simulink model "Test_Sistema_piero"  (R2022b)
settings: Solver=VariableStepAuto  StartTime=0.0  StopTime=10.0  RelTol=1e-3
libraries: arduinolib x11, simulink x3
settings Model: Creator=marqu  LastModifiedBy=marqu

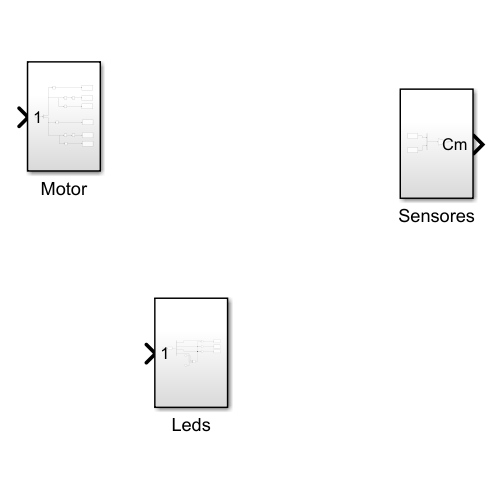
[thumbnail: Simulink's stored preview of the top-level diagram]
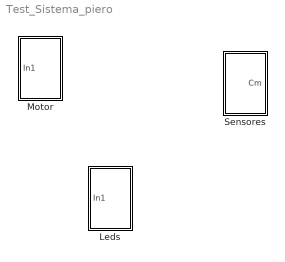
== system Test_Sistema_piero ==
  Leds : Subsystem
  Motor : Subsystem
  Sensores : Subsystem

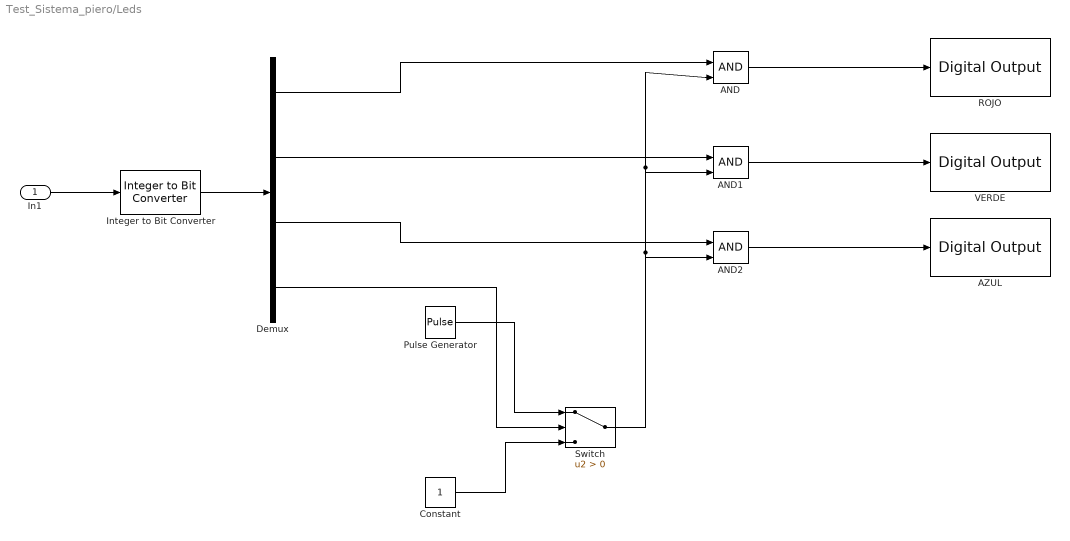
== system Test_Sistema_piero/Leds ==
  In1 : Inport
  AND : Logic  IconShape=distinctive  AllPortsSameDT=off  OutDataTypeStr=boolean
  AND1 : Logic  IconShape=distinctive  AllPortsSameDT=off  OutDataTypeStr=boolean
  AND2 : Logic  IconShape=distinctive  AllPortsSameDT=off  OutDataTypeStr=boolean
  AZUL : arduinolib/Digital Output  pinNumber=53  Direction=output  blockPlatform=arduino
  Constant : Constant
  Demux : Demux
  Integer to Bit Converter : simulink/Logic and Bit Operations/Integer to Bit Converter  nbits=3  signedInputValues=Unsigned  bitOrder=MSB first  outDtype=Inherit via internal rule
  Pulse Generator : DiscretePulseGenerator  PulseType=Time based  Period=10  PulseWidth=5
  ROJO : arduinolib/Digital Output  pinNumber=49  Direction=output  blockPlatform=arduino
  Switch : Switch  Criteria=u2 > Threshold  SaturateOnIntegerOverflow=off  InputSameDT=off
  VERDE : arduinolib/Digital Output  pinNumber=51  Direction=output  blockPlatform=arduino
  wires:
  AND1/1 -> VERDE/1
  Demux/4 -> Switch/2
  Integer to Bit Converter/1 -> Demux/1
  Constant/1 -> Switch/3
  Demux/3 -> AND2/1
  Demux/1 -> AND/1
  Demux/2 -> AND1/1
  Switch/1 -> AND2/2, AND1/2, AND/2
  AND2/1 -> AZUL/1
  In1/1 -> Integer to Bit Converter/1
  AND/1 -> ROJO/1
  Pulse Generator/1 -> Switch/1

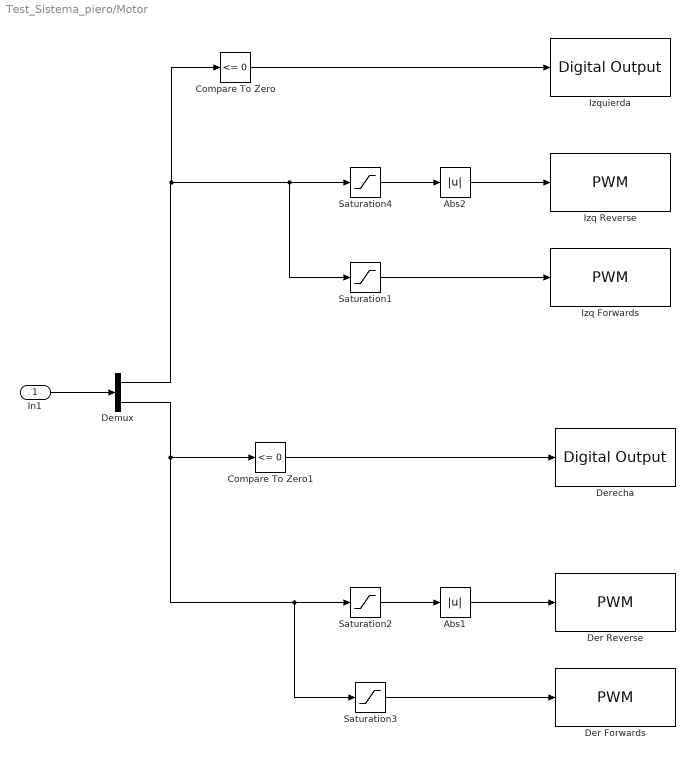
== system Test_Sistema_piero/Motor ==
  In1 : Inport
  Abs1 : Abs  SaturateOnIntegerOverflow=off
  Abs2 : Abs  SaturateOnIntegerOverflow=off
  Compare To Zero : simulink/Logic and Bit Operations/Compare To Zero  relop=<=  OutDataTypeStr=boolean
  Compare To Zero1 : simulink/Logic and Bit Operations/Compare To Zero  relop=<=  OutDataTypeStr=boolean
  Demux : Demux  Outputs=2
  Der Forwards : arduinolib/PWM  pinNumber=11  frequencyType=Default  desiredFrequency=490.2  achievableFrequency=490.2
  Der Reverse : arduinolib/PWM  pinNumber=12  frequencyType=Default  desiredFrequency=490.2  achievableFrequency=490.2
  Derecha : arduinolib/Digital Output  pinNumber=13  Direction=output  blockPlatform=arduino
  Izq Forwards : arduinolib/PWM  pinNumber=10  frequencyType=Default  desiredFrequency=490.2  achievableFrequency=490.2
  Izq Reverse : arduinolib/PWM  pinNumber=9  frequencyType=Default  desiredFrequency=490.2  achievableFrequency=490.2
  Izquierda : arduinolib/Digital Output  pinNumber=8  Direction=output  blockPlatform=arduino
  Saturation{1..4} (4 alike) : Saturate
  wires:
  In1/1 -> Demux/1
  Abs1/1 -> Der Reverse/1
  Compare To Zero1/1 -> Derecha/1
  Abs2/1 -> Izq Reverse/1
  Compare To Zero/1 -> Izquierda/1
  Demux/1 -> Compare To Zero/1, Saturation4/1, Saturation1/1
  Demux/2 -> Compare To Zero1/1, Saturation2/1, Saturation3/1
  Saturation3/1 -> Der Forwards/1
  Saturation4/1 -> Abs2/1
  Saturation1/1 -> Izq Forwards/1
  Saturation2/1 -> Abs1/1

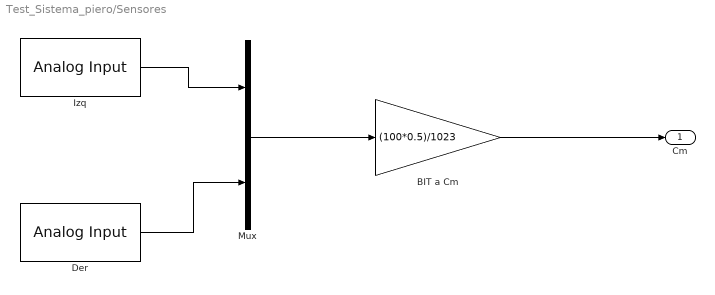
== system Test_Sistema_piero/Sensores ==
  BIT a Cm : Gain  Gain=(100*0.5)/1023
  Der : arduinolib/Analog Input  pinNumber=4  ReadResultsOnly=off  ConversionTriggerSource=Software  ExternalTriggerType=uint32( 0 )  OutputDataType=uint16  EnableConversionCompleteNotify=off  EnableOuputStatus=off  SampleTime=-1  blockPlatform=arduino
  Izq : arduinolib/Analog Input  pinNumber=4  ReadResultsOnly=off  ConversionTriggerSource=Software  ExternalTriggerType=uint32( 0 )  OutputDataType=uint16  EnableConversionCompleteNotify=off  EnableOuputStatus=off  SampleTime=-1  blockPlatform=arduino
  Mux : Mux  Inputs=2
  Cm : Outport
  wires:
  BIT a Cm/1 -> Cm/1
  Der/1 -> Mux/2
  Izq/1 -> Mux/1
  Mux/1 -> BIT a Cm/1
